simulink model "YXXRJFPID"  (Simulink 8.3)
settings: Solver=ode4  SolverMode=SingleTasking  StartTime=0.0  StopTime=1  FixedStep=0.001  RelTol=1e-3
undefined symbols (not defined in the file or in its folder): DiscIntNeverNeededParam
settings Model: Creator=Zhu Supeng  LastModifiedBy=Zhu Supeng
settings DataIOCC: SignalLoggingName=sigsOut
settings DebuggingCC: SaveWithParameterizedLinksMsg=none  SignalResolutionControl=TryResolveAllWithWarning  SolverPrmCheckMsg=none  MultiTaskDSMMsg=warning  MultiTaskCondExecSysMsg=none  StateNameClashWarn=none
settings HardwareCC: TargetUnknown=on
settings RTWCC: IncludeERTFirstTime=on

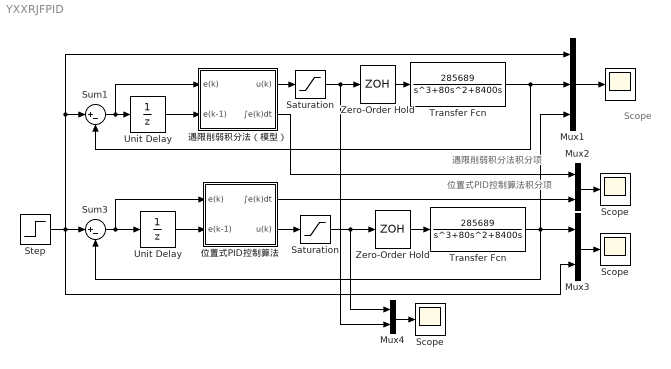
== system YXXRJFPID ==
  note: 位置式PID控制算法积分项
  note: 遇限削弱积分法积分项
  note: Scope
  " " : Scope
      settings: YMin=0  YMax=50  SaveName=YXXRJFPID  MaxDataPoints=500000
  " Scope " : Scope
      settings: YMin=0  YMax=1.8  SaveName=YXXRJFPIDu  MaxDataPoints=500000
  Mux1 : Mux  Inputs=3
  Mux2 : Mux  Inputs=2
  Mux3 : Mux  Inputs=2
  Mux4 : Mux  Inputs=2
  Saturation : Saturate  UpperLimit=10  LowerLimit=-10
  "Saturation  " : Saturate  UpperLimit=10  LowerLimit=-10
  Scope : Scope
      settings: YMin=0  YMax=50  SaveName=ScopeData6  MaxDataPoints=500000
  "Scope " : Scope
      settings: YMin=0  YMax=1.8  SaveName=YXXRJFPIDI  MaxDataPoints=500000
  Step : Step  Time=0  After=30  SampleTime=0
  Sum1 : Sum  Inputs=|+-  SaturateOnIntegerOverflow=on
  Sum3 : Sum  Inputs=|+-  SaturateOnIntegerOverflow=on
  "Transfer Fcn " : TransferFcn  Numerator=[285689]  Denominator="[1 80  8400 0]"
  "Transfer Fcn  " : TransferFcn  Numerator=[285689]  Denominator="[1 80  8400 0]"
  Unit Delay : UnitDelay  SampleTime=0.001
  "Unit Delay  " : UnitDelay  SampleTime=0.001
  Zero-Order Hold : ZeroOrderHold  SampleTime=0.001
  "Zero-Order Hold " : ZeroOrderHold  SampleTime=0.001
  位置式PID控制算法 : Subsystem
  遇限削弱积分法（模型） : Subsystem
  wires:
  位置式PID控制算法/2(u(k)) -> "Saturation  "/1
  Zero-Order Hold/1 -> "Transfer Fcn  "/1
  "Transfer Fcn  "/1 -> Sum3/2, Mux3/1, Mux1/3
  Unit Delay/1 -> 位置式PID控制算法/2(e(k-1))
  Mux3/1 -> Scope/1
  Step/1 -> Sum3/1, Sum1/1, Mux1/1, Mux3/2
  遇限削弱积分法（模型）/1(u(k)) -> Saturation/1
  "Zero-Order Hold "/1 -> "Transfer Fcn "/1
  "Transfer Fcn "/1 -> Mux1/2, Sum1/2
  "Unit Delay  "/1 -> 遇限削弱积分法（模型）/2(e(k-1))
  Mux1/1 -> " "/1
  Mux2/1 -> "Scope "/1
  位置式PID控制算法/1(∫e(k)dt) -> Mux2/2
  遇限削弱积分法（模型）/2(∫e(k)dt) -> Mux2/1
  Saturation/1 -> "Zero-Order Hold "/1, Mux4/2
  Sum3/1 -> Unit Delay/1, 位置式PID控制算法/1(e(k))
  "Saturation  "/1 -> Zero-Order Hold/1, Mux4/1
  Sum1/1 -> "Unit Delay  "/1, 遇限削弱积分法（模型）/1(e(k))
  Mux4/1 -> " Scope "/1

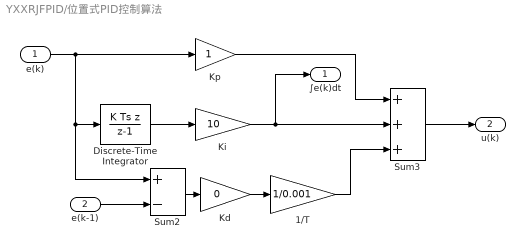
== system YXXRJFPID/位置式PID控制算法 ==
  e(k) : Inport
  e(k-1) : Inport  Port=2
  1/T : Gain  Gain=1/0.001  SaturateOnIntegerOverflow=on  OutDataTypeStr=Inherit: Same as input  ParamDataTypeStr=Inherit: Same as input
  Discrete-Time Integrator : DiscreteIntegrator  IntegratorMethod=Integration: Backward Euler  SampleTime=0.001  ICPrevOutput=DiscIntNeverNeededParam  ICPrevScaledInput=DiscIntNeverNeededParam
  Kd : Gain  Gain=0  SaturateOnIntegerOverflow=on  OutDataTypeStr=Inherit: Same as input  ParamDataTypeStr=Inherit: Same as input
  Ki : Gain  Gain=10  SaturateOnIntegerOverflow=on  OutDataTypeStr=Inherit: Same as input  ParamDataTypeStr=Inherit: Same as input
  Kp : Gain  SaturateOnIntegerOverflow=on  OutDataTypeStr=Inherit: Same as input  ParamDataTypeStr=Inherit: Same as input
  Sum2 : Sum  Inputs=+-  SaturateOnIntegerOverflow=on
  Sum3 : Sum  Inputs=+++  SaturateOnIntegerOverflow=on
  ∫e(k)dt : Outport
  u(k) : Outport  Port=2
  wires:
  Ki/1 -> Sum3/2, ∫e(k)dt/1
  1/T/1 -> Sum3/3
  e(k-1)/1 -> Sum2/2
  Discrete-Time Integrator/1 -> Ki/1
  Kd/1 -> 1/T/1
  Sum3/1 -> u(k)/1
  Kp/1 -> Sum3/1
  e(k)/1 -> Sum2/1, Discrete-Time Integrator/1, Kp/1
  Sum2/1 -> Kd/1

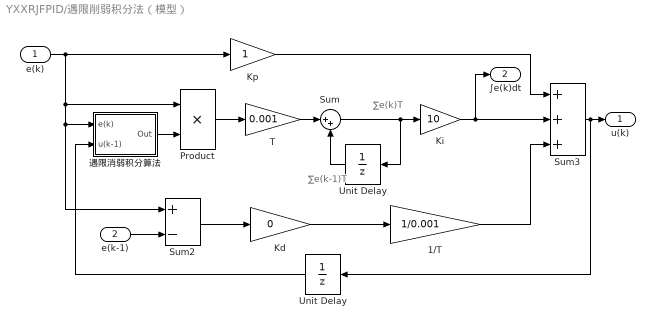
== system YXXRJFPID/遇限削弱积分法（模型） ==
  note: ∑e(k)T
  note: ∑e(k-1)T
  e(k) : Inport
  e(k-1) : Inport  Port=2
  1/T : Gain  Gain=1/0.001  SaturateOnIntegerOverflow=on  OutDataTypeStr=Inherit: Same as input  ParamDataTypeStr=Inherit: Same as input
  Kd : Gain  Gain=0  SaturateOnIntegerOverflow=on  OutDataTypeStr=Inherit: Same as input  ParamDataTypeStr=Inherit: Same as input
  Ki : Gain  Gain=10  SaturateOnIntegerOverflow=on  OutDataTypeStr=Inherit: Same as input  ParamDataTypeStr=Inherit: Same as input
  Kp : Gain  SaturateOnIntegerOverflow=on  OutDataTypeStr=Inherit: Same as input  ParamDataTypeStr=Inherit: Same as input
  Product : Product  SaturateOnIntegerOverflow=on  OutDataTypeStr=Inherit: Same as first input
  Sum : Sum  Inputs=|++  SaturateOnIntegerOverflow=on
  Sum2 : Sum  Inputs=+-  SaturateOnIntegerOverflow=on
  Sum3 : Sum  Inputs=+++  SaturateOnIntegerOverflow=on
  T : Gain  Gain=0.001  SaturateOnIntegerOverflow=on  OutDataTypeStr=Inherit: Same as input  ParamDataTypeStr=Inherit: Same as input
  Unit Delay : UnitDelay  SampleTime=0.001
  "Unit Delay " : UnitDelay  SampleTime=0.001
  遇限消弱积分算法 : Subsystem
  u(k) : Outport
  ∫e(k)dt : Outport  Port=2
  wires:
  Sum2/1 -> Kd/1
  e(k)/1 -> Kp/1, Product/1, Sum2/1, 遇限消弱积分算法/1(e(k))
  Kp/1 -> Sum3/1
  Sum3/1 -> Unit Delay/1, u(k)/1
  Kd/1 -> 1/T/1
  e(k-1)/1 -> Sum2/2
  1/T/1 -> Sum3/3
  遇限消弱积分算法/1("Out ") -> Product/2
  Ki/1 -> Sum3/2, ∫e(k)dt/1
  Unit Delay/1 -> 遇限消弱积分算法/2(u(k-1))
  Sum/1 -> "Unit Delay "/1, Ki/1
  "Unit Delay "/1 -> Sum/2
  T/1 -> Sum/1
  Product/1 -> T/1

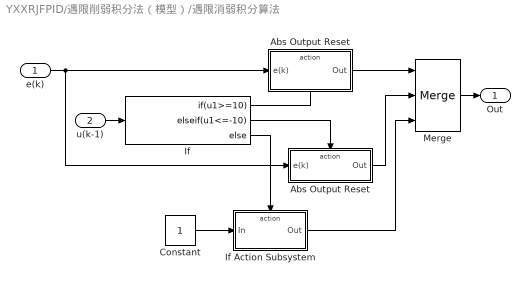
== system YXXRJFPID/遇限削弱积分法（模型）/遇限消弱积分算法 ==
  e(k) : Inport
  u(k-1) : Inport  Port=2
  Abs Output Reset : Subsystem  TreatAsAtomicUnit=on
  "Abs Output Reset " : Subsystem  TreatAsAtomicUnit=on
  Constant : Constant
  If : If  IfExpression=u1>=10  ElseIfExpressions=u1<=-10
  If Action Subsystem : Subsystem  TreatAsAtomicUnit=on
  Merge : Merge  Inputs=3
  "Out " : Outport
  wires:
  u(k-1)/1 -> If/1
  Merge/1 -> "Out "/1
  If/1 -> Abs Output Reset/Action
  e(k)/1 -> Abs Output Reset/1(e(k)), "Abs Output Reset "/1(e(k))
  If/2 -> "Abs Output Reset "/Action
  Abs Output Reset/1(Out) -> Merge/1
  "Abs Output Reset "/1(Out) -> Merge/2
  If/3 -> If Action Subsystem/Action
  Constant/1 -> If Action Subsystem/1(In)
  If Action Subsystem/1(Out) -> Merge/3

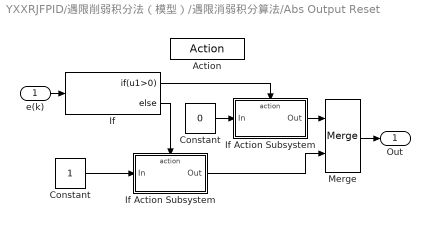
== system YXXRJFPID/遇限削弱积分法（模型）/遇限消弱积分算法/Abs Output Reset ==
  e(k) : Inport
  Action : ActionPort  InitializeStates=reset  ActionType=then
  Constant : Constant  Value=0
  "Constant " : Constant
  If : If  IfExpression=u1>0
  If Action Subsystem : Subsystem  TreatAsAtomicUnit=on
  "If Action Subsystem " : Subsystem  TreatAsAtomicUnit=on
  Merge : Merge
  Out : Outport  OutputWhenDisabled=reset  InitialOutput=0
  wires:
  e(k)/1 -> If/1
  Constant/1 -> If Action Subsystem/1(In)
  If Action Subsystem/1(Out) -> Merge/1
  "Constant "/1 -> "If Action Subsystem "/1(In)
  If/2 -> "If Action Subsystem "/Action
  "If Action Subsystem "/1(Out) -> Merge/2
  Merge/1 -> Out/1
  If/1 -> If Action Subsystem/Action

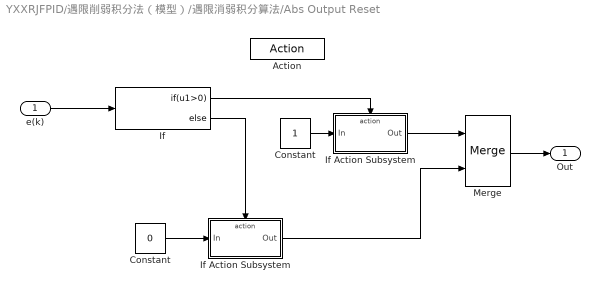
== system YXXRJFPID/遇限削弱积分法（模型）/遇限消弱积分算法/Abs Output Reset  ==
  e(k) : Inport
  Action : ActionPort  InitializeStates=reset  ActionType=elseif
  Constant : Constant
  "Constant " : Constant  Value=0
  If : If  IfExpression=u1>0
  If Action Subsystem : Subsystem  TreatAsAtomicUnit=on
  "If Action Subsystem " : Subsystem  TreatAsAtomicUnit=on
  Merge : Merge
  Out : Outport  OutputWhenDisabled=reset  InitialOutput=0
  wires:
  Merge/1 -> Out/1
  "If Action Subsystem "/1(Out) -> Merge/2
  If/2 -> "If Action Subsystem "/Action
  "Constant "/1 -> "If Action Subsystem "/1(In)
  If Action Subsystem/1(Out) -> Merge/1
  Constant/1 -> If Action Subsystem/1(In)
  e(k)/1 -> If/1
  If/1 -> If Action Subsystem/Action

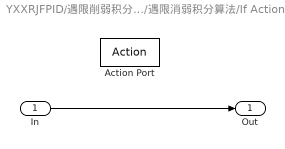
== system YXXRJFPID/遇限削弱积分法（模型）/遇限消弱积分算法/If Action Subsystem ==
  In : Inport
  Action Port : ActionPort  ActionType=else
  Out : Outport
  wires:
  In/1 -> Out/1

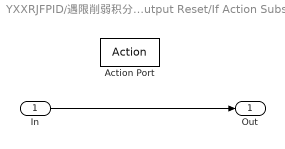
== system YXXRJFPID/遇限削弱积分法（模型）/遇限消弱积分算法/Abs Output Reset/If Action Subsystem ==
  In : Inport
  Action Port : ActionPort  ActionType=then
  Out : Outport
  wires:
  In/1 -> Out/1

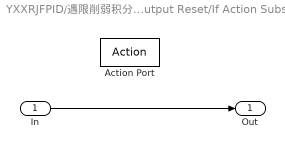
== system YXXRJFPID/遇限削弱积分法（模型）/遇限消弱积分算法/Abs Output Reset/If Action Subsystem  ==
  In : Inport
  Action Port : ActionPort  ActionType=else
  Out : Outport
  wires:
  In/1 -> Out/1

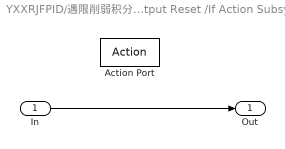
== system YXXRJFPID/遇限削弱积分法（模型）/遇限消弱积分算法/Abs Output Reset /If Action Subsystem ==
  In : Inport
  Action Port : ActionPort  ActionType=then
  Out : Outport
  wires:
  In/1 -> Out/1

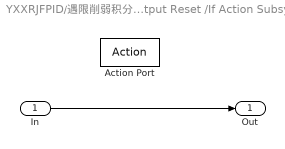
== system YXXRJFPID/遇限削弱积分法（模型）/遇限消弱积分算法/Abs Output Reset /If Action Subsystem  ==
  In : Inport
  Action Port : ActionPort  ActionType=else
  Out : Outport
  wires:
  In/1 -> Out/1
